simulink model "labcomp"  (R2017b)
settings: Solver=VariableStepAuto  StartTime=0.0  StopTime=50  RelTol=1e-3
settings Model: Creator=miguel  LastModifiedBy=miguel

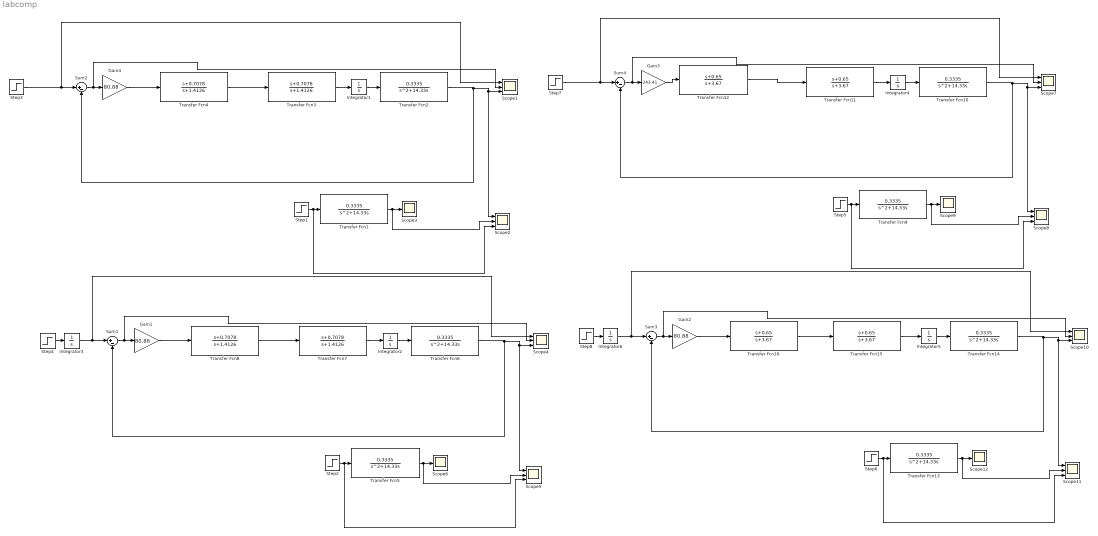
== system labcomp ==
  Gain1 : Gain  Gain=80.88
  Gain2 : Gain  Gain=80.88
  Gain3 : Gain  Gain=243.41
  Gain4 : Gain  Gain=80.88
  Integrator{1..6} (6 alike) : Integrator
  Scope{1..2,4..5,7..8,10..11} (8 alike) : Scope  NumInputPorts=3
  Scope{3,6,9,12} (4 alike) : Scope
  Step{1..8} (8 alike) : Step  SampleTime=0
  Sum{1..4} (4 alike) : Sum  Inputs=|+-
  Transfer Fcn{1..2,5..6,9..10,13..14} (8 alike) : TransferFcn  Numerator=[0.3335 ]  Denominator=[1 14.33 0]
  Transfer Fcn{11..12,15..16} (4 alike) : TransferFcn  Numerator=[1 0.65]  Denominator=[1 3.67]
  Transfer Fcn{3..4,7..8} (4 alike) : TransferFcn  Numerator=[1 0.7078]  Denominator=[1 1.4126]
  wires:
  Step1/1 -> Transfer Fcn1/1, Scope2/3
  Sum2/1 -> Gain4/1, Scope1/2
  Step3/1 -> Sum2/1, Scope1/1
  Transfer Fcn2/1 -> Sum2/2, Scope1/3, Scope2/1
  Integrator1/1 -> Transfer Fcn2/1
  Transfer Fcn1/1 -> Scope3/1, Scope2/2
  Transfer Fcn3/1 -> Integrator1/1
  Gain4/1 -> Transfer Fcn4/1
  Transfer Fcn4/1 -> Transfer Fcn3/1
  Transfer Fcn8/1 -> Transfer Fcn7/1
  Gain1/1 -> Transfer Fcn8/1
  Transfer Fcn7/1 -> Integrator2/1
  Transfer Fcn5/1 -> Scope5/2, Scope6/1
  Integrator2/1 -> Transfer Fcn6/1
  Transfer Fcn6/1 -> Scope5/1, Scope4/3, Sum1/2
  Step4/1 -> Integrator3/1
  Sum1/1 -> Scope4/2, Gain1/1
  Step2/1 -> Scope5/3, Transfer Fcn5/1
  Integrator3/1 -> Scope4/1, Sum1/1
  Integrator6/1 -> Sum3/1, Scope10/1
  Step6/1 -> Transfer Fcn13/1, Scope11/3
  Sum3/1 -> Gain2/1, Scope10/2
  Step8/1 -> Integrator6/1
  Transfer Fcn14/1 -> Sum3/2, Scope10/3, Scope11/1
  Integrator5/1 -> Transfer Fcn14/1
  Transfer Fcn13/1 -> Scope12/1, Scope11/2
  Transfer Fcn15/1 -> Integrator5/1
  Gain2/1 -> Transfer Fcn16/1
  Transfer Fcn12/1 -> Transfer Fcn11/1
  Gain3/1 -> Transfer Fcn12/1
  Transfer Fcn11/1 -> Integrator4/1
  Transfer Fcn9/1 -> Scope8/2, Scope9/1
  Integrator4/1 -> Transfer Fcn10/1
  Transfer Fcn10/1 -> Scope8/1, Scope7/3, Sum4/2
  Step7/1 -> Scope7/1, Sum4/1
  Sum4/1 -> Scope7/2, Gain3/1
  Step5/1 -> Scope8/3, Transfer Fcn9/1
  Transfer Fcn16/1 -> Transfer Fcn15/1
